simulink model "Q11"  (Simulink 7.9)
settings: Solver=ode45  StartTime=0.0  StopTime=10.0  RelTol=1e-3
settings Model: Creator=ramit  LastModifiedBy=ramit

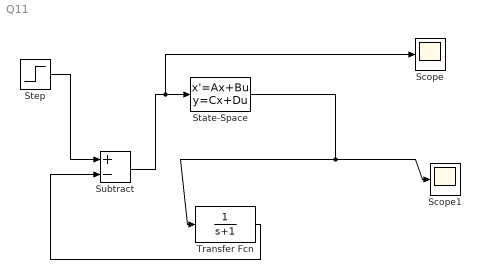
== system Q11 ==
  Scope : Scope
  Scope1 : Scope
  State-Space : StateSpace  A="[-2  -1;1 0]"  B=[1;0]  C=[1 0]  D=0
  Step : Step  SampleTime=0
  Subtract : Sum  Inputs=+-
  Transfer Fcn : TransferFcn  Denominator=[1 1]
  wires:
  Step/1 -> Subtract/1
  Subtract/1 -> State-Space/1, Scope/1
  State-Space/1 -> Transfer Fcn/1, Scope1/1
  Transfer Fcn/1 -> Subtract/2
